simulink model "sudoku_PP_CEX2"  (R2017b)
settings: Solver=FixedStepDiscrete  StartTime=0.0  StopTime=10.0  FixedStep=0.200000  RelTol=1e-3
model workspace (MAT data in the model file):
  ContractValidatorBlocksMap = containers.Map
  ContractValidatorBlocksMap.serialization.keys = {'sudoku/contract/validator'}
  ContractValidatorBlocksMap.serialization.values{1}.block = 'sudoku/contract/validator'
  ContractValidatorBlocksMap.serialization.values{1}.assumePorts = 1
  ContractValidatorBlocksMap.serialization.values{1}.guaranteePorts = 1
  ContractValidatorBlocksMap.serialization.values{1}.modeBlocksPorts = 0
  ContractValidatorBlocksMap.serialization.values{1}.portHandles.Inport = [423.005737305 424.004150391]
  ContractValidatorBlocksMap.serialization.values{1}.portHandles.Outport = 425.013793945
  ContractValidatorBlocksMap.serialization.values{1}.portHandles.Enable = []
  ContractValidatorBlocksMap.serialization.values{1}.portHandles.Trigger = []
  ContractValidatorBlocksMap.serialization.values{1}.portHandles.State = []
  ContractValidatorBlocksMap.serialization.values{1}.portHandles.LConn = []
  ContractValidatorBlocksMap.serialization.values{1}.portHandles.RConn = []
  ContractValidatorBlocksMap.serialization.values{1}.portHandles.Ifaction = []
  ContractValidatorBlocksMap.serialization.values{1}.portHandles.Reset = []
  ContractValidatorBlocksMap.serialization.values{1}.portConnectivity(1).Type = '1'
  ContractValidatorBlocksMap.serialization.values{1}.portConnectivity(1).Position = [385 130]
  ContractValidatorBlocksMap.serialization.values{1}.portConnectivity(1).SrcBlock = 97.0111083984
  ContractValidatorBlocksMap.serialization.values{1}.portConnectivity(1).SrcPort = 0
  ContractValidatorBlocksMap.serialization.values{1}.portConnectivity(1).DstBlock = []
  ContractValidatorBlocksMap.serialization.values{1}.portConnectivity(1).DstPort = []
  ContractValidatorBlocksMap.serialization.values{1}.portConnectivity(2).Type = '2'
  ContractValidatorBlocksMap.serialization.values{1}.portConnectivity(2).Position = [385 270]
  ContractValidatorBlocksMap.serialization.values{1}.portConnectivity(2).SrcBlock = 134.024414062
  ContractValidatorBlocksMap.serialization.values{1}.portConnectivity(2).SrcPort = 0
  ContractValidatorBlocksMap.serialization.values{1}.portConnectivity(2).DstBlock = []
  ContractValidatorBlocksMap.serialization.values{1}.portConnectivity(2).DstPort = []
  ContractValidatorBlocksMap.serialization.values{1}.portConnectivity(3).Type = '1'
  ContractValidatorBlocksMap.serialization.values{1}.portConnectivity(3).Position = [500 200]
  ContractValidatorBlocksMap.serialization.values{1}.portConnectivity(3).SrcBlock = []
  ContractValidatorBlocksMap.serialization.values{1}.portConnectivity(3).SrcPort = []
  ContractValidatorBlocksMap.serialization.values{1}.portConnectivity(3).DstBlock = 409.010986328
  ContractValidatorBlocksMap.serialization.values{1}.portConnectivity(3).DstPort = 0
  ContractValidatorBlocksMap.serialization.uniformity = 0
  ContractValidatorBlocksMap.serialization.keyType = 'char'
  ContractValidatorBlocksMap.serialization.valueType = 'any'
  already_pp = 1
  compositionalMap.analysisNames = {'sudoku_PP/Sudoku'}
  compositionalMap.compositionalOptions = {{''}}
  compositionalMap.selectedOptions = 1
  maskControlsMap = containers.Map
  maskControlsMap.serialization.keys = {'sudoku_PP/contract/guarantee'}
  maskControlsMap.serialization.values = {{'Display_counter_example_as_signals', 'Display_counter_example_as_tables', 'Display_counter_example_as_HTML_tables', 'Generate_an_outer_model_for_the_counter_example', 'Generate_an_inner_model_for_the_counter_example'}}
  maskControlsMap.serialization.uniformity = 0
  maskControlsMap.serialization.keyType = 'char'
  maskControlsMap.serialization.valueType = 'any'
  nodeNameToBlockNameMap : containers.Map (value not decoded)
  verificationResults : struct (value not decoded)
undefined symbols (not defined in the file): contractAfterSimulation, ContractAssumeBlock, contractBeforeSimulation, ContractBlock, ContractGuaranteeBlock, ContractValidatorBlock, saveValidatorParameters
(part 1 of 17)
settings Model: Creator=hbourbou  LastModifiedBy=hbourbou
settings DebuggingCC: AlgebraicLoopMsg=error  ArtificialAlgebraicLoopMsg=error  SingleTaskRateTransMsg=error

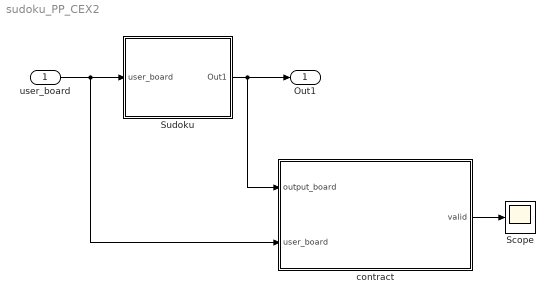
== system sudoku_PP_CEX2 ==
  user_board : Inport  OutDataTypeStr=uint8  PortDimensions=[9,9]
  Scope : Scope
  Sudoku : Subsystem  TreatAsAtomicUnit=on
  contract : Subsystem  TreatAsAtomicUnit=on  mask(ContractBlock){ContractBlockType=ContractBlock}
      mask init:
      | set_param(gcb, 'LinkStatus', 'none');
      settings: CopyFcn=set_param(gcb, 'LinkStatus', 'none');
      mask DialogControl DescTextVar Prompt: Contract block
      mask Display:
      | text(0.5, 0.5, '{\bf\fontsize{20}Contract}', 'hor', 'center', 'texmode','on');
      | blocks = find_system(gcb, 'LookUnderMasks','all', 'SearchDepth',1,'BlockType','Inport');
      | for i = 1 : length(blocks)
      |     blockName = get_param(blocks(i), 'Name');
      |     [path, blockName] = fileparts(char(blockName));
      |     port_label('input', i, blockName);
      | end
      | 
      | blocks = find_system(gcb, 'LookUnderMasks','all', 'SearchDepth',1,'BlockType','Outport');
      | for i = 1 : length(blocks)
      |     blockName = get_param(blocks(i), 'Name');
      |     [path, blockName] = fileparts(char(blockName));
      |     port_label('output', i, blockName);
      | end
  Out1 : Outport
  wires:
  Sudoku/1(Out1) -> contract/1(output_board), Out1/1
  user_board/1 -> contract/2(user_board), Sudoku/1(user_board)
  contract/1(valid) -> Scope/1

== system sudoku_PP_CEX2/Sudoku ==
  user_board : Inport
  Sum : Sum  Inputs=|++
  initial_board1 : Constant  Value=[0 0 0 0 0 0 0 0 0; 0 0 0 0 0 3 0 8 5; 0 0 1 0 2 0 0 0 0; 0 0 0 5 0 7 0 0 0; 0 0 4 0 0 0 1 0 0; 0 9 0 0 0 0 0 0 0; 5 0 0 0 0 0 0 7 3; 0 0 2 0 1 0 0 0 0; 0 0 0 0 4 0 0 0 9]  OutDataTypeStr=uint8
  Out1 : Outport
  wires:
  user_board/1 -> Sum/2
  initial_board1/1 -> Sum/1
  Sum/1 -> Out1/1

== system sudoku_PP_CEX2/contract ==
  output_board : Inport
  user_board : Inport  Port=2
  assume : Subsystem  TreatAsAtomicUnit=on  mask(ContractAssumeBlock){ContractBlockType=ContractAssumeBlock}
      mask init:
      | set_param(gcb, 'LinkStatus', 'none');
      mask DialogControl DescTextVar Prompt: Assume block
  guarantee : Subsystem  TreatAsAtomicUnit=on  mask(ContractGuaranteeBlock){ContractBlockType=ContractGuaranteeBlock}
      mask init:
      | set_param(gcb, 'LinkStatus', 'none');
      mask DialogControl DescTextVar Prompt: Guarantee block
      mask DialogControl Display_counter_example_as_signals Prompt: Display counter example as signals
      mask DialogControl Display_counter_example_as_signals Callback: displayCexSignals(1, 1);
      mask DialogControl Display_counter_example_as_tables Prompt: Display counter example as tables
      mask DialogControl Display_counter_example_as_tables Callback: displayCexTables(1, 1);
      mask DialogControl Display_counter_example_as_HTML_tables Prompt: Display counter example as HTML tables
      mask DialogControl Display_counter_example_as_HTML_tables Callback: displayCexHtmlTables(1, 1);
      mask DialogControl Generate_an_outer_model_for_the_counter_example Prompt: Generate an outer model for the counter example
      mask DialogControl Generate_an_outer_model_for_the_counter_example Callback: generateModelWithSignalBuilders(1, 1, 2);
      mask DialogControl Generate_an_inner_model_for_the_counter_example Prompt: Generate an inner model for the counter example
      mask DialogControl Generate_an_inner_model_for_the_counter_example Callback: generateModelWithSignalBuilders(1, 1, 1);
  validator : M-S-Function  LoadFcn=saveValidatorParameters(gcb);  InitFcn=contractBeforeSimulation();  StopFcn=contractAfterSimulation();  FunctionName=contract  mask(ContractValidatorBlock){assumePorts=1, guaranteePorts=1, modePorts=0, ContractBlockType=ContractValidatorBlock, createInportsCheckbox=off}
      mask prompts: assumePorts "Assume ports     :"; guaranteePorts "Guarantee ports :"; modePorts "Mode ports        :"; createInportsCheckbox "Create inports and connect them automatically"
      mask init:
      | set_param(gcb,'LinkStatus','none');
      | contract_callback('inputs_callback',gcb);
      mask DialogControl DescTextVar Prompt: The validator block implements the following logic: <br> <br> <b>Sofar</b>(assume<sub>1</sub> <b>&#8743;</b> assume<sub>2</sub> <b>&#8743;</b> ... assume<sub>k</sub>) <b>&rarr;</b> (guarantee<sub>1</sub> <b>&#8743;</b> guarantee<sub>2</sub> <b>&#8743;</b> ... guarantee<sub>m</sub> <b>&#8743;</b>  mode<sub>1</sub> <b>&#8743;</b> mode<sub>2</sub> <b>&#8743;</b> ... <b>&#8743;</b> mode<sub>n</sub> )<br> where mode<sub>i</sub> = require<sub>i</sub> <b>&rarr;</b> ensure<sub>i</sub>
      mask Display:
      | color('black');
      | port_label('input',1,'assume');
      | port_label('input',2,'guarantee');
      | port_label('output',1,'valid');
  valid : Outport
  wires:
  output_board/1 -> guarantee/1(Board)
  validator/1 -> valid/1
  guarantee/1(guarantee) -> validator/2
  assume/1(assume) -> validator/1
  user_board/1 -> assume/1(board)

== system sudoku_PP_CEX2/contract/assume ==
  board : Inport
  Element_minus_Wise_newline_Product : Product
  Logical_newline_Operator : Logic  Inputs=1  AllPortsSameDT=off  OutDataTypeStr=boolean
  Relational_newline_Operator : RelationalOperator  Operator===  OutDataTypeStr=boolean  RndMeth=Simplest
  Reshape : Reshape
  initial_board : Constant  Value=[0 0 0 0 0 0 0 0 0; 0 0 0 0 0 3 0 8 5; 0 0 1 0 2 0 0 0 0; 0 0 0 5 0 7 0 0 0; 0 0 4 0 0 0 1 0 0; 0 9 0 0 0 0 0 0 0; 5 0 0 0 0 0 0 7 3; 0 0 2 0 1 0 0 0 0; 0 0 0 0 4 0 0 0 9]  OutDataTypeStr=uint8
  zero : Constant  Value=zeros(9,9)  OutDataTypeStr=uint8
  assume : Outport  OutDataTypeStr=boolean
  wires:
  initial_board/1 -> Element_minus_Wise_newline_Product/1
  board/1 -> Element_minus_Wise_newline_Product/2
  Element_minus_Wise_newline_Product/1 -> Relational_newline_Operator/1
  zero/1 -> Relational_newline_Operator/2
  Relational_newline_Operator/1 -> Reshape/1
  Logical_newline_Operator/1 -> assume/1
  Reshape/1 -> Logical_newline_Operator/1

== system sudoku_PP_CEX2/contract/guarantee ==
  Board : Inport  PortDimensions=[9 9]
  BoxesValid : Subsystem  TreatAsAtomicUnit=on
  ColsValid : Subsystem  TreatAsAtomicUnit=on
  Logical_newline_Operator : Logic  Inputs=3  AllPortsSameDT=off  OutDataTypeStr=boolean
  Logical_newline_Operator1 : Logic  Operator=NOT  AllPortsSameDT=off  OutDataTypeStr=boolean
  RowsValid : Subsystem  TreatAsAtomicUnit=on
  guarantee : Outport  OutDataTypeStr=boolean
  wires:
  Board/1 -> BoxesValid/1(In1), RowsValid/1(In1), ColsValid/1(In1)
  RowsValid/1(Out1) -> Logical_newline_Operator/1
  ColsValid/1(Out1) -> Logical_newline_Operator/2
  BoxesValid/1(Out1) -> Logical_newline_Operator/3
  Logical_newline_Operator/1 -> Logical_newline_Operator1/1
  Logical_newline_Operator1/1 -> guarantee/1

== system sudoku_PP_CEX2/contract/guarantee/BoxesValid ==
  In1 : Inport
  ForEach_newline_Subsystem : Subsystem  TreatAsAtomicUnit=on
  Logical_newline_Operator : Logic  Inputs=1  AllPortsSameDT=off  OutDataTypeStr=boolean
  Out1 : Outport
  wires:
  In1/1 -> ForEach_newline_Subsystem/1(In1)
  ForEach_newline_Subsystem/1(Out1) -> Logical_newline_Operator/1
  Logical_newline_Operator/1 -> Out1/1

== system sudoku_PP_CEX2/contract/guarantee/ColsValid ==
  In1 : Inport
  ForEach_newline_Subsystem : Subsystem  TreatAsAtomicUnit=on
  Logical_newline_Operator : Logic  Inputs=1  AllPortsSameDT=off  OutDataTypeStr=boolean
  Out1 : Outport
  wires:
  In1/1 -> ForEach_newline_Subsystem/1(In1)
  ForEach_newline_Subsystem/1(Out1) -> Logical_newline_Operator/1
  Logical_newline_Operator/1 -> Out1/1

== system sudoku_PP_CEX2/contract/guarantee/RowsValid ==
  In1 : Inport
  ForEach_newline_Subsystem : Subsystem  TreatAsAtomicUnit=on
  Logical_newline_Operator : Logic  Inputs=1  AllPortsSameDT=off  OutDataTypeStr=boolean
  Out1 : Outport
  wires:
  In1/1 -> ForEach_newline_Subsystem/1(In1)
  ForEach_newline_Subsystem/1(Out1) -> Logical_newline_Operator/1
  Logical_newline_Operator/1 -> Out1/1

== system sudoku_PP_CEX2/contract/guarantee/BoxesValid/ForEach_newline_Subsystem ==
  In1 : Inport
  Concatenate_1 : Concatenate  NumInputs=3  Mode=Multidimensional array
  ForEach1 : Subsystem  TreatAsAtomicUnit=on
  ForEach2 : Subsystem  TreatAsAtomicUnit=on
  ForEach3 : Subsystem  TreatAsAtomicUnit=on
  Selector_1_In1 : Selector  NumberOfDimensions=2  IndexOptions=Index vector (dialog),Select all  Indices=[1 2 3],  OutputSizes=1
  Selector_2_In1 : Selector  NumberOfDimensions=2  IndexOptions=Index vector (dialog),Select all  Indices=[4 5 6],  OutputSizes=1
  Selector_3_In1 : Selector  NumberOfDimensions=2  IndexOptions=Index vector (dialog),Select all  Indices=[7 8 9],  OutputSizes=1
  Out1 : Outport
  wires:
  Concatenate_1/1 -> Out1/1
  Selector_3_In1/1 -> ForEach3/1(In1)
  Selector_2_In1/1 -> ForEach2/1(In1)
  Selector_1_In1/1 -> ForEach1/1(In1)
  ForEach3/1(Out1) -> Concatenate_1/3
  ForEach2/1(Out1) -> Concatenate_1/2
  ForEach1/1(Out1) -> Concatenate_1/1
  In1/1 -> Selector_3_In1/1, Selector_2_In1/1, Selector_1_In1/1

== system sudoku_PP_CEX2/contract/guarantee/ColsValid/ForEach_newline_Subsystem ==
  In1 : Inport
  Concatenate_1 : Concatenate  NumInputs=9  Mode=Multidimensional array
  ForEach1 : Subsystem  TreatAsAtomicUnit=on
  ForEach2 : Subsystem  TreatAsAtomicUnit=on
  ForEach3 : Subsystem  TreatAsAtomicUnit=on
  ForEach4 : Subsystem  TreatAsAtomicUnit=on
  ForEach5 : Subsystem  TreatAsAtomicUnit=on
  ForEach6 : Subsystem  TreatAsAtomicUnit=on
  ForEach7 : Subsystem  TreatAsAtomicUnit=on
  ForEach8 : Subsystem  TreatAsAtomicUnit=on
  ForEach9 : Subsystem  TreatAsAtomicUnit=on
  Selector_1_In1 : Selector  NumberOfDimensions=2  IndexOptions=Select all,Index vector (dialog)  Indices=,1  OutputSizes=1
  Selector_2_In1 : Selector  NumberOfDimensions=2  IndexOptions=Select all,Index vector (dialog)  Indices=,2  OutputSizes=1
  Selector_3_In1 : Selector  NumberOfDimensions=2  IndexOptions=Select all,Index vector (dialog)  Indices=,3  OutputSizes=1
  Selector_4_In1 : Selector  NumberOfDimensions=2  IndexOptions=Select all,Index vector (dialog)  Indices=,4  OutputSizes=1
  Selector_5_In1 : Selector  NumberOfDimensions=2  IndexOptions=Select all,Index vector (dialog)  Indices=,5  OutputSizes=1
  Selector_6_In1 : Selector  NumberOfDimensions=2  IndexOptions=Select all,Index vector (dialog)  Indices=,6  OutputSizes=1
  Selector_7_In1 : Selector  NumberOfDimensions=2  IndexOptions=Select all,Index vector (dialog)  Indices=,7  OutputSizes=1
  Selector_8_In1 : Selector  NumberOfDimensions=2  IndexOptions=Select all,Index vector (dialog)  Indices=,8  OutputSizes=1
  Selector_9_In1 : Selector  NumberOfDimensions=2  IndexOptions=Select all,Index vector (dialog)  Indices=,9  OutputSizes=1
  Out1 : Outport
  wires:
  Concatenate_1/1 -> Out1/1
  Selector_9_In1/1 -> ForEach9/1(In1)
  Selector_8_In1/1 -> ForEach8/1(In1)
  Selector_7_In1/1 -> ForEach7/1(In1)
  Selector_6_In1/1 -> ForEach6/1(In1)
  Selector_5_In1/1 -> ForEach5/1(In1)
  Selector_4_In1/1 -> ForEach4/1(In1)
  Selector_3_In1/1 -> ForEach3/1(In1)
  Selector_2_In1/1 -> ForEach2/1(In1)
  Selector_1_In1/1 -> ForEach1/1(In1)
  ForEach9/1(Out1) -> Concatenate_1/9
  ForEach8/1(Out1) -> Concatenate_1/8
  ForEach7/1(Out1) -> Concatenate_1/7
  ForEach6/1(Out1) -> Concatenate_1/6
  ForEach5/1(Out1) -> Concatenate_1/5
  ForEach4/1(Out1) -> Concatenate_1/4
  ForEach3/1(Out1) -> Concatenate_1/3
  ForEach2/1(Out1) -> Concatenate_1/2
  ForEach1/1(Out1) -> Concatenate_1/1
  In1/1 -> Selector_9_In1/1, Selector_8_In1/1, Selector_7_In1/1, Selector_6_In1/1, Selector_5_In1/1, Selector_4_In1/1, Selector_3_In1/1, Selector_2_In1/1, Selector_1_In1/1

== system sudoku_PP_CEX2/contract/guarantee/RowsValid/ForEach_newline_Subsystem ==
  In1 : Inport
  Concatenate_1 : Concatenate  NumInputs=9  Mode=Multidimensional array
  ForEach1 : Subsystem  TreatAsAtomicUnit=on
  ForEach2 : Subsystem  TreatAsAtomicUnit=on
  ForEach3 : Subsystem  TreatAsAtomicUnit=on
  ForEach4 : Subsystem  TreatAsAtomicUnit=on
  ForEach5 : Subsystem  TreatAsAtomicUnit=on
  ForEach6 : Subsystem  TreatAsAtomicUnit=on
  ForEach7 : Subsystem  TreatAsAtomicUnit=on
  ForEach8 : Subsystem  TreatAsAtomicUnit=on
  ForEach9 : Subsystem  TreatAsAtomicUnit=on
  Selector_1_In1 : Selector  NumberOfDimensions=2  IndexOptions=Index vector (dialog),Select all  Indices=1,  OutputSizes=1
  Selector_2_In1 : Selector  NumberOfDimensions=2  IndexOptions=Index vector (dialog),Select all  Indices=2,  OutputSizes=1
  Selector_3_In1 : Selector  NumberOfDimensions=2  IndexOptions=Index vector (dialog),Select all  Indices=3,  OutputSizes=1
  Selector_4_In1 : Selector  NumberOfDimensions=2  IndexOptions=Index vector (dialog),Select all  Indices=4,  OutputSizes=1
  Selector_5_In1 : Selector  NumberOfDimensions=2  IndexOptions=Index vector (dialog),Select all  Indices=5,  OutputSizes=1
  Selector_6_In1 : Selector  NumberOfDimensions=2  IndexOptions=Index vector (dialog),Select all  Indices=6,  OutputSizes=1
  Selector_7_In1 : Selector  NumberOfDimensions=2  IndexOptions=Index vector (dialog),Select all  Indices=7,  OutputSizes=1
  Selector_8_In1 : Selector  NumberOfDimensions=2  IndexOptions=Index vector (dialog),Select all  Indices=8,  OutputSizes=1
  Selector_9_In1 : Selector  NumberOfDimensions=2  IndexOptions=Index vector (dialog),Select all  Indices=9,  OutputSizes=1
  Out1 : Outport
  wires:
  Concatenate_1/1 -> Out1/1
  Selector_9_In1/1 -> ForEach9/1(In1)
  Selector_8_In1/1 -> ForEach8/1(In1)
  Selector_7_In1/1 -> ForEach7/1(In1)
  Selector_6_In1/1 -> ForEach6/1(In1)
  Selector_5_In1/1 -> ForEach5/1(In1)
  Selector_4_In1/1 -> ForEach4/1(In1)
  Selector_3_In1/1 -> ForEach3/1(In1)
  Selector_2_In1/1 -> ForEach2/1(In1)
  Selector_1_In1/1 -> ForEach1/1(In1)
  ForEach9/1(Out1) -> Concatenate_1/9
  ForEach8/1(Out1) -> Concatenate_1/8
  ForEach7/1(Out1) -> Concatenate_1/7
  ForEach6/1(Out1) -> Concatenate_1/6
  ForEach5/1(Out1) -> Concatenate_1/5
  ForEach4/1(Out1) -> Concatenate_1/4
  ForEach3/1(Out1) -> Concatenate_1/3
  ForEach2/1(Out1) -> Concatenate_1/2
  ForEach1/1(Out1) -> Concatenate_1/1
  In1/1 -> Selector_9_In1/1, Selector_8_In1/1, Selector_7_In1/1, Selector_6_In1/1, Selector_5_In1/1, Selector_4_In1/1, Selector_3_In1/1, Selector_2_In1/1, Selector_1_In1/1

== system sudoku_PP_CEX2/contract/guarantee/BoxesValid/ForEach_newline_Subsystem/ForEach1 ==
  In1 : Inport
  ForEach_newline_Subsystem : Subsystem  TreatAsAtomicUnit=on
  Logical_newline_Operator : Logic  Inputs=1  AllPortsSameDT=off  OutDataTypeStr=boolean
  Out1 : Outport
  wires:
  Logical_newline_Operator/1 -> Out1/1
  ForEach_newline_Subsystem/1(Out1) -> Logical_newline_Operator/1
  In1/1 -> ForEach_newline_Subsystem/1(In1)

== system sudoku_PP_CEX2/contract/guarantee/BoxesValid/ForEach_newline_Subsystem/ForEach2 ==
  In1 : Inport
  ForEach_newline_Subsystem : Subsystem  TreatAsAtomicUnit=on
  Logical_newline_Operator : Logic  Inputs=1  AllPortsSameDT=off  OutDataTypeStr=boolean
  Out1 : Outport
  wires:
  Logical_newline_Operator/1 -> Out1/1
  ForEach_newline_Subsystem/1(Out1) -> Logical_newline_Operator/1
  In1/1 -> ForEach_newline_Subsystem/1(In1)

== system sudoku_PP_CEX2/contract/guarantee/BoxesValid/ForEach_newline_Subsystem/ForEach3 ==
  In1 : Inport
  ForEach_newline_Subsystem : Subsystem  TreatAsAtomicUnit=on
  Logical_newline_Operator : Logic  Inputs=1  AllPortsSameDT=off  OutDataTypeStr=boolean
  Out1 : Outport
  wires:
  Logical_newline_Operator/1 -> Out1/1
  ForEach_newline_Subsystem/1(Out1) -> Logical_newline_Operator/1
  In1/1 -> ForEach_newline_Subsystem/1(In1)

== system sudoku_PP_CEX2/contract/guarantee/ColsValid/ForEach_newline_Subsystem/ForEach1 ==
  In1 : Inport
  Vectorisvalid : Subsystem  TreatAsAtomicUnit=on
  Out1 : Outport
  wires:
  Vectorisvalid/1(Out1) -> Out1/1
  In1/1 -> Vectorisvalid/1(In1)

== system sudoku_PP_CEX2/contract/guarantee/ColsValid/ForEach_newline_Subsystem/ForEach2 ==
  In1 : Inport
  Vectorisvalid : Subsystem  TreatAsAtomicUnit=on
  Out1 : Outport
  wires:
  Vectorisvalid/1(Out1) -> Out1/1
  In1/1 -> Vectorisvalid/1(In1)

== system sudoku_PP_CEX2/contract/guarantee/ColsValid/ForEach_newline_Subsystem/ForEach3 ==
  In1 : Inport
  Vectorisvalid : Subsystem  TreatAsAtomicUnit=on
  Out1 : Outport
  wires:
  Vectorisvalid/1(Out1) -> Out1/1
  In1/1 -> Vectorisvalid/1(In1)

== system sudoku_PP_CEX2/contract/guarantee/ColsValid/ForEach_newline_Subsystem/ForEach4 ==
  In1 : Inport
  Vectorisvalid : Subsystem  TreatAsAtomicUnit=on
  Out1 : Outport
  wires:
  Vectorisvalid/1(Out1) -> Out1/1
  In1/1 -> Vectorisvalid/1(In1)

== system sudoku_PP_CEX2/contract/guarantee/ColsValid/ForEach_newline_Subsystem/ForEach5 ==
  In1 : Inport
  Vectorisvalid : Subsystem  TreatAsAtomicUnit=on
  Out1 : Outport
  wires:
  Vectorisvalid/1(Out1) -> Out1/1
  In1/1 -> Vectorisvalid/1(In1)

== system sudoku_PP_CEX2/contract/guarantee/ColsValid/ForEach_newline_Subsystem/ForEach6 ==
  In1 : Inport
  Vectorisvalid : Subsystem  TreatAsAtomicUnit=on
  Out1 : Outport
  wires:
  Vectorisvalid/1(Out1) -> Out1/1
  In1/1 -> Vectorisvalid/1(In1)

== system sudoku_PP_CEX2/contract/guarantee/ColsValid/ForEach_newline_Subsystem/ForEach7 ==
  In1 : Inport
  Vectorisvalid : Subsystem  TreatAsAtomicUnit=on
  Out1 : Outport
  wires:
  Vectorisvalid/1(Out1) -> Out1/1
  In1/1 -> Vectorisvalid/1(In1)

== system sudoku_PP_CEX2/contract/guarantee/ColsValid/ForEach_newline_Subsystem/ForEach8 ==
  In1 : Inport
  Vectorisvalid : Subsystem  TreatAsAtomicUnit=on
  Out1 : Outport
  wires:
  Vectorisvalid/1(Out1) -> Out1/1
  In1/1 -> Vectorisvalid/1(In1)

== system sudoku_PP_CEX2/contract/guarantee/ColsValid/ForEach_newline_Subsystem/ForEach9 ==
  In1 : Inport
  Vectorisvalid : Subsystem  TreatAsAtomicUnit=on
  Out1 : Outport
  wires:
  Vectorisvalid/1(Out1) -> Out1/1
  In1/1 -> Vectorisvalid/1(In1)

== system sudoku_PP_CEX2/contract/guarantee/RowsValid/ForEach_newline_Subsystem/ForEach1 ==
  In1 : Inport
  Vectorisvalid : Subsystem  TreatAsAtomicUnit=on
  Out1 : Outport
  wires:
  Vectorisvalid/1(Out1) -> Out1/1
  In1/1 -> Vectorisvalid/1(In1)

== system sudoku_PP_CEX2/contract/guarantee/RowsValid/ForEach_newline_Subsystem/ForEach2 ==
  In1 : Inport
  Vectorisvalid : Subsystem  TreatAsAtomicUnit=on
  Out1 : Outport
  wires:
  Vectorisvalid/1(Out1) -> Out1/1
  In1/1 -> Vectorisvalid/1(In1)

== system sudoku_PP_CEX2/contract/guarantee/RowsValid/ForEach_newline_Subsystem/ForEach3 ==
  In1 : Inport
  Vectorisvalid : Subsystem  TreatAsAtomicUnit=on
  Out1 : Outport
  wires:
  Vectorisvalid/1(Out1) -> Out1/1
  In1/1 -> Vectorisvalid/1(In1)

== system sudoku_PP_CEX2/contract/guarantee/RowsValid/ForEach_newline_Subsystem/ForEach4 ==
  In1 : Inport
  Vectorisvalid : Subsystem  TreatAsAtomicUnit=on
  Out1 : Outport
  wires:
  Vectorisvalid/1(Out1) -> Out1/1
  In1/1 -> Vectorisvalid/1(In1)

== system sudoku_PP_CEX2/contract/guarantee/RowsValid/ForEach_newline_Subsystem/ForEach5 ==
  In1 : Inport
  Vectorisvalid : Subsystem  TreatAsAtomicUnit=on
  Out1 : Outport
  wires:
  Vectorisvalid/1(Out1) -> Out1/1
  In1/1 -> Vectorisvalid/1(In1)

== system sudoku_PP_CEX2/contract/guarantee/RowsValid/ForEach_newline_Subsystem/ForEach6 ==
  In1 : Inport
  Vectorisvalid : Subsystem  TreatAsAtomicUnit=on
  Out1 : Outport
  wires:
  Vectorisvalid/1(Out1) -> Out1/1
  In1/1 -> Vectorisvalid/1(In1)

== system sudoku_PP_CEX2/contract/guarantee/RowsValid/ForEach_newline_Subsystem/ForEach7 ==
  In1 : Inport
  Vectorisvalid : Subsystem  TreatAsAtomicUnit=on
  Out1 : Outport
  wires:
  Vectorisvalid/1(Out1) -> Out1/1
  In1/1 -> Vectorisvalid/1(In1)

== system sudoku_PP_CEX2/contract/guarantee/RowsValid/ForEach_newline_Subsystem/ForEach8 ==
  In1 : Inport
  Vectorisvalid : Subsystem  TreatAsAtomicUnit=on
  Out1 : Outport
  wires:
  Vectorisvalid/1(Out1) -> Out1/1
  In1/1 -> Vectorisvalid/1(In1)

== system sudoku_PP_CEX2/contract/guarantee/RowsValid/ForEach_newline_Subsystem/ForEach9 ==
  In1 : Inport
  Vectorisvalid : Subsystem  TreatAsAtomicUnit=on
  Out1 : Outport
  wires:
  Vectorisvalid/1(Out1) -> Out1/1
  In1/1 -> Vectorisvalid/1(In1)

== system sudoku_PP_CEX2/contract/guarantee/BoxesValid/ForEach_newline_Subsystem/ForEach1/ForEach_newline_Subsystem ==
  In1 : Inport
  Concatenate_1 : Concatenate  NumInputs=3  Mode=Multidimensional array
  ForEach1 : Subsystem  TreatAsAtomicUnit=on
  ForEach2 : Subsystem  TreatAsAtomicUnit=on
  ForEach3 : Subsystem  TreatAsAtomicUnit=on
  Selector_1_In1 : Selector  NumberOfDimensions=2  IndexOptions=Select all,Index vector (dialog)  Indices=,[1 2 3]  OutputSizes=1
  Selector_2_In1 : Selector  NumberOfDimensions=2  IndexOptions=Select all,Index vector (dialog)  Indices=,[4 5 6]  OutputSizes=1
  Selector_3_In1 : Selector  NumberOfDimensions=2  IndexOptions=Select all,Index vector (dialog)  Indices=,[7 8 9]  OutputSizes=1
  Out1 : Outport
  wires:
  Concatenate_1/1 -> Out1/1
  Selector_3_In1/1 -> ForEach3/1(In1)
  Selector_2_In1/1 -> ForEach2/1(In1)
  Selector_1_In1/1 -> ForEach1/1(In1)
  ForEach3/1(Out1) -> Concatenate_1/3
  ForEach2/1(Out1) -> Concatenate_1/2
  ForEach1/1(Out1) -> Concatenate_1/1
  In1/1 -> Selector_3_In1/1, Selector_2_In1/1, Selector_1_In1/1

== system sudoku_PP_CEX2/contract/guarantee/BoxesValid/ForEach_newline_Subsystem/ForEach2/ForEach_newline_Subsystem ==
  In1 : Inport
  Concatenate_1 : Concatenate  NumInputs=3  Mode=Multidimensional array
  ForEach1 : Subsystem  TreatAsAtomicUnit=on
  ForEach2 : Subsystem  TreatAsAtomicUnit=on
  ForEach3 : Subsystem  TreatAsAtomicUnit=on
  Selector_1_In1 : Selector  NumberOfDimensions=2  IndexOptions=Select all,Index vector (dialog)  Indices=,[1 2 3]  OutputSizes=1
  Selector_2_In1 : Selector  NumberOfDimensions=2  IndexOptions=Select all,Index vector (dialog)  Indices=,[4 5 6]  OutputSizes=1
  Selector_3_In1 : Selector  NumberOfDimensions=2  IndexOptions=Select all,Index vector (dialog)  Indices=,[7 8 9]  OutputSizes=1
  Out1 : Outport
  wires:
  Concatenate_1/1 -> Out1/1
  Selector_3_In1/1 -> ForEach3/1(In1)
  Selector_2_In1/1 -> ForEach2/1(In1)
  Selector_1_In1/1 -> ForEach1/1(In1)
  ForEach3/1(Out1) -> Concatenate_1/3
  ForEach2/1(Out1) -> Concatenate_1/2
  ForEach1/1(Out1) -> Concatenate_1/1
  In1/1 -> Selector_3_In1/1, Selector_2_In1/1, Selector_1_In1/1

== system sudoku_PP_CEX2/contract/guarantee/BoxesValid/ForEach_newline_Subsystem/ForEach3/ForEach_newline_Subsystem ==
  In1 : Inport
  Concatenate_1 : Concatenate  NumInputs=3  Mode=Multidimensional array
  ForEach1 : Subsystem  TreatAsAtomicUnit=on
  ForEach2 : Subsystem  TreatAsAtomicUnit=on
  ForEach3 : Subsystem  TreatAsAtomicUnit=on
  Selector_1_In1 : Selector  NumberOfDimensions=2  IndexOptions=Select all,Index vector (dialog)  Indices=,[1 2 3]  OutputSizes=1
  Selector_2_In1 : Selector  NumberOfDimensions=2  IndexOptions=Select all,Index vector (dialog)  Indices=,[4 5 6]  OutputSizes=1
  Selector_3_In1 : Selector  NumberOfDimensions=2  IndexOptions=Select all,Index vector (dialog)  Indices=,[7 8 9]  OutputSizes=1
  Out1 : Outport
  wires:
  Concatenate_1/1 -> Out1/1
  Selector_3_In1/1 -> ForEach3/1(In1)
  Selector_2_In1/1 -> ForEach2/1(In1)
  Selector_1_In1/1 -> ForEach1/1(In1)
  ForEach3/1(Out1) -> Concatenate_1/3
  ForEach2/1(Out1) -> Concatenate_1/2
  ForEach1/1(Out1) -> Concatenate_1/1
  In1/1 -> Selector_3_In1/1, Selector_2_In1/1, Selector_1_In1/1

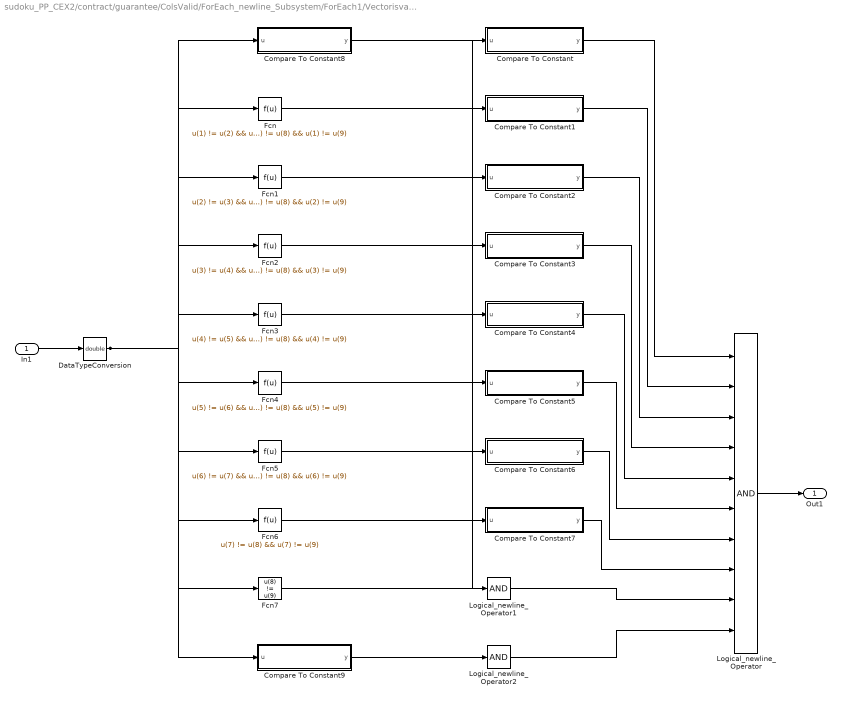
== system sudoku_PP_CEX2/contract/guarantee/ColsValid/ForEach_newline_Subsystem/ForEach1/Vectorisvalid ==
  In1 : Inport
  Compare To Constant : Subsystem  AncestorBlock=|  TreatAsAtomicUnit=on  mask(Compare To Constant){relop===, const=1, OutDataTypeStr=boolean, ZeroCross=on}
      | simulink/Logic and Bit
      | Operations/Compare
      | To Constant
      mask prompts: relop "Simulink:masks:Operator_MP"; const "Simulink:masks:ConstantValue_MP"; OutDataTypeStr "Simulink:masks:OutputDataType_MP"; ZeroCross "Simulink:masks:EnableZerocrossingDetection_MP"
      mask help: Simulink:masks:CompareToConstant_MD
      mask init:
      | blkName = gcb;
      | 
      | if strcmp(get_param(gcbh,'OutDataTypeStr'),'boolean')
      | 	setValue = 'boolean';
      | else
      | 	setValue = 'fixdt(0, 8)';
      | end
      | 
      | set_param([blkName,'/Compare'],'relop',relop, ...
      | 	'OutDataTypeStr', setValue, 'ZeroCross', ZeroCross);
      | 
      | str = [relop,' C']; %default
      | 
      | const_str = get_param(blkName, 'const');
      | const_val = str2num(const_str);
      | 
      | if isempty(const_val) %#ok<ST2NM>
      |     %Expression/Variable
      |     str = [relop, ' ', strtrim(const_str)];
      | else
      |     if length(const_val) == 1 
      |         if Simulink.data.isSupportedEnumClass(class(const_val))
      |             % Special Handling for Enumerations
      |             if Simulink.data.getEnumTypeInfo(class(const_val), 'AddClassNameToEnumNames')
      |                 str = [relop, ' ', strtrim(const_str)];
      |             else
      |                 str = [relop, ' ', char(const_val)];
      |             end
      |         elseif(isfloat(const_val) || isinteger(const_val) || islogical(const_val)) 
      |                 str = [relop, ' ', num2str(const_val)];
      |         end
      |     end
      | end
      mask TypeOptions relop: == | ~= | < | <= | >= | >
      mask TypeOptions OutDataTypeStr: Simulink:masks:uint8 | Simulink:masks:boolean
      mask Callback ZeroCross: sl('zeroCrossEnable', gcbh);
      mask Display: disp(str)
  Compare To Constant1 : Subsystem  AncestorBlock=|  TreatAsAtomicUnit=on  mask(Compare To Constant){relop===, const=1, OutDataTypeStr=boolean, ZeroCross=on}
      | simulink/Logic and Bit
      | Operations/Compare
      | To Constant
      mask prompts: relop "Simulink:masks:Operator_MP"; const "Simulink:masks:ConstantValue_MP"; OutDataTypeStr "Simulink:masks:OutputDataType_MP"; ZeroCross "Simulink:masks:EnableZerocrossingDetection_MP"
      mask help: Simulink:masks:CompareToConstant_MD
      mask init: same as sudoku_PP_CEX2/contract/guarantee/ColsValid/ForEach_newline_Subsystem/ForEach1/Vectorisvalid/Compare To Constant
      mask TypeOptions relop: == | ~= | < | <= | >= | >
      mask TypeOptions OutDataTypeStr: Simulink:masks:uint8 | Simulink:masks:boolean
      mask Callback ZeroCross: sl('zeroCrossEnable', gcbh);
      mask Display: disp(str)
  Compare To Constant2 : Subsystem  AncestorBlock=|  TreatAsAtomicUnit=on  mask(Compare To Constant){relop===, const=1, OutDataTypeStr=boolean, ZeroCross=on}
      | simulink/Logic and Bit
      | Operations/Compare
      | To Constant
      mask prompts: relop "Simulink:masks:Operator_MP"; const "Simulink:masks:ConstantValue_MP"; OutDataTypeStr "Simulink:masks:OutputDataType_MP"; ZeroCross "Simulink:masks:EnableZerocrossingDetection_MP"
      mask help: Simulink:masks:CompareToConstant_MD
      mask init: same as sudoku_PP_CEX2/contract/guarantee/ColsValid/ForEach_newline_Subsystem/ForEach1/Vectorisvalid/Compare To Constant
      mask TypeOptions relop: == | ~= | < | <= | >= | >
      mask TypeOptions OutDataTypeStr: Simulink:masks:uint8 | Simulink:masks:boolean
      mask Callback ZeroCross: sl('zeroCrossEnable', gcbh);
      mask Display: disp(str)
  Compare To Constant3 : Subsystem  AncestorBlock=|  TreatAsAtomicUnit=on  mask(Compare To Constant){relop===, const=1, OutDataTypeStr=boolean, ZeroCross=on}
      | simulink/Logic and Bit
      | Operations/Compare
      | To Constant
      mask prompts: relop "Simulink:masks:Operator_MP"; const "Simulink:masks:ConstantValue_MP"; OutDataTypeStr "Simulink:masks:OutputDataType_MP"; ZeroCross "Simulink:masks:EnableZerocrossingDetection_MP"
      mask help: Simulink:masks:CompareToConstant_MD
      mask init: same as sudoku_PP_CEX2/contract/guarantee/ColsValid/ForEach_newline_Subsystem/ForEach1/Vectorisvalid/Compare To Constant
      mask TypeOptions relop: == | ~= | < | <= | >= | >
      mask TypeOptions OutDataTypeStr: Simulink:masks:uint8 | Simulink:masks:boolean
      mask Callback ZeroCross: sl('zeroCrossEnable', gcbh);
      mask Display: disp(str)
  Compare To Constant4 : Subsystem  AncestorBlock=|  TreatAsAtomicUnit=on  mask(Compare To Constant){relop===, const=1, OutDataTypeStr=boolean, ZeroCross=on}
      | simulink/Logic and Bit
      | Operations/Compare
      | To Constant
      mask prompts: relop "Simulink:masks:Operator_MP"; const "Simulink:masks:ConstantValue_MP"; OutDataTypeStr "Simulink:masks:OutputDataType_MP"; ZeroCross "Simulink:masks:EnableZerocrossingDetection_MP"
      mask help: Simulink:masks:CompareToConstant_MD
      mask init: same as sudoku_PP_CEX2/contract/guarantee/ColsValid/ForEach_newline_Subsystem/ForEach1/Vectorisvalid/Compare To Constant
      mask TypeOptions relop: == | ~= | < | <= | >= | >
      mask TypeOptions OutDataTypeStr: Simulink:masks:uint8 | Simulink:masks:boolean
      mask Callback ZeroCross: sl('zeroCrossEnable', gcbh);
      mask Display: disp(str)
  Compare To Constant5 : Subsystem  AncestorBlock=|  TreatAsAtomicUnit=on  mask(Compare To Constant){relop===, const=1, OutDataTypeStr=boolean, ZeroCross=on}
      | simulink/Logic and Bit
      | Operations/Compare
      | To Constant
      mask prompts: relop "Simulink:masks:Operator_MP"; const "Simulink:masks:ConstantValue_MP"; OutDataTypeStr "Simulink:masks:OutputDataType_MP"; ZeroCross "Simulink:masks:EnableZerocrossingDetection_MP"
      mask help: Simulink:masks:CompareToConstant_MD
      mask init: same as sudoku_PP_CEX2/contract/guarantee/ColsValid/ForEach_newline_Subsystem/ForEach1/Vectorisvalid/Compare To Constant
      mask TypeOptions relop: == | ~= | < | <= | >= | >
      mask TypeOptions OutDataTypeStr: Simulink:masks:uint8 | Simulink:masks:boolean
      mask Callback ZeroCross: sl('zeroCrossEnable', gcbh);
      mask Display: disp(str)
  Compare To Constant6 : Subsystem  AncestorBlock=|  TreatAsAtomicUnit=on  mask(Compare To Constant){relop===, const=1, OutDataTypeStr=boolean, ZeroCross=on}
      | simulink/Logic and Bit
      | Operations/Compare
      | To Constant
      mask prompts: relop "Simulink:masks:Operator_MP"; const "Simulink:masks:ConstantValue_MP"; OutDataTypeStr "Simulink:masks:OutputDataType_MP"; ZeroCross "Simulink:masks:EnableZerocrossingDetection_MP"
      mask help: Simulink:masks:CompareToConstant_MD
      mask init: same as sudoku_PP_CEX2/contract/guarantee/ColsValid/ForEach_newline_Subsystem/ForEach1/Vectorisvalid/Compare To Constant
      mask TypeOptions relop: == | ~= | < | <= | >= | >
      mask TypeOptions OutDataTypeStr: Simulink:masks:uint8 | Simulink:masks:boolean
      mask Callback ZeroCross: sl('zeroCrossEnable', gcbh);
      mask Display: disp(str)
  Compare To Constant7 : Subsystem  AncestorBlock=|  TreatAsAtomicUnit=on  mask(Compare To Constant){relop===, const=1, OutDataTypeStr=boolean, ZeroCross=on}
      | simulink/Logic and Bit
      | Operations/Compare
      | To Constant
      mask prompts: relop "Simulink:masks:Operator_MP"; const "Simulink:masks:ConstantValue_MP"; OutDataTypeStr "Simulink:masks:OutputDataType_MP"; ZeroCross "Simulink:masks:EnableZerocrossingDetection_MP"
      mask help: Simulink:masks:CompareToConstant_MD
      mask init: same as sudoku_PP_CEX2/contract/guarantee/ColsValid/ForEach_newline_Subsystem/ForEach1/Vectorisvalid/Compare To Constant
      mask TypeOptions relop: == | ~= | < | <= | >= | >
      mask TypeOptions OutDataTypeStr: Simulink:masks:uint8 | Simulink:masks:boolean
      mask Callback ZeroCross: sl('zeroCrossEnable', gcbh);
      mask Display: disp(str)
  Compare To Constant8 : Subsystem  AncestorBlock=|  TreatAsAtomicUnit=on  mask(Compare To Constant){relop=>=, const=1, OutDataTypeStr=boolean, ZeroCross=on}
      | simulink/Logic and Bit
      | Operations/Compare
      | To Constant
      mask prompts: relop "Simulink:masks:Operator_MP"; const "Simulink:masks:ConstantValue_MP"; OutDataTypeStr "Simulink:masks:OutputDataType_MP"; ZeroCross "Simulink:masks:EnableZerocrossingDetection_MP"
      mask help: Simulink:masks:CompareToConstant_MD
      mask init: same as sudoku_PP_CEX2/contract/guarantee/ColsValid/ForEach_newline_Subsystem/ForEach1/Vectorisvalid/Compare To Constant
      mask TypeOptions relop: == | ~= | < | <= | >= | >
      mask TypeOptions OutDataTypeStr: Simulink:masks:uint8 | Simulink:masks:boolean
      mask Callback ZeroCross: sl('zeroCrossEnable', gcbh);
      mask Display: disp(str)
  Compare To Constant9 : Subsystem  AncestorBlock=|  TreatAsAtomicUnit=on  mask(Compare To Constant){relop=<=, const=9, OutDataTypeStr=boolean, ZeroCross=on}
      | simulink/Logic and Bit
      | Operations/Compare
      | To Constant
      mask prompts: relop "Simulink:masks:Operator_MP"; const "Simulink:masks:ConstantValue_MP"; OutDataTypeStr "Simulink:masks:OutputDataType_MP"; ZeroCross "Simulink:masks:EnableZerocrossingDetection_MP"
      mask help: Simulink:masks:CompareToConstant_MD
      mask init: same as sudoku_PP_CEX2/contract/guarantee/ColsValid/ForEach_newline_Subsystem/ForEach1/Vectorisvalid/Compare To Constant
      mask TypeOptions relop: == | ~= | < | <= | >= | >
      mask TypeOptions OutDataTypeStr: Simulink:masks:uint8 | Simulink:masks:boolean
      mask Callback ZeroCross: sl('zeroCrossEnable', gcbh);
      mask Display: disp(str)
  DataTypeConversion : DataTypeConversion  OutDataTypeStr=double
  Fcn : Fcn  Expr=u(1) != u(2) && u(1) != u(3) && u(1) != u(4) && u(1) != u(5) && u(1) != u(6) && u(1) != u(7) && u(1) != u(8) && u(1) != u(9)
  Fcn1 : Fcn  Expr=u(2) != u(3) && u(2) != u(4) && u(2) != u(5) && u(2) != u(6) && u(2) != u(7) && u(2) != u(8) && u(2) != u(9)
  Fcn2 : Fcn  Expr=u(3) != u(4) && u(3) != u(5) && u(3) != u(6) && u(3) != u(7) && u(3) != u(8) && u(3) != u(9)
  Fcn3 : Fcn  Expr=u(4) != u(5) && u(4) != u(6) && u(4) != u(7) && u(4) != u(8) && u(4) != u(9)
  Fcn4 : Fcn  Expr=u(5) != u(6) && u(5) != u(7) && u(5) != u(8) && u(5) != u(9)
  Fcn5 : Fcn  Expr=u(6) != u(7) && u(6) != u(8) && u(6) != u(9)
  Fcn6 : Fcn  Expr=u(7) != u(8) && u(7) != u(9)
  Fcn7 : Fcn  Expr=u(8) != u(9)
  Logical_newline_Operator : Logic  Inputs=10  AllPortsSameDT=off  OutDataTypeStr=boolean
  Logical_newline_Operator1 : Logic  Inputs=1  AllPortsSameDT=off  OutDataTypeStr=boolean
  Logical_newline_Operator2 : Logic  Inputs=1  AllPortsSameDT=off  OutDataTypeStr=boolean
  Out1 : Outport
  wires:
  Logical_newline_Operator/1 -> Out1/1
  Compare To Constant9/1(y) -> Logical_newline_Operator2/1
  Compare To Constant8/1(y) -> Logical_newline_Operator1/1
  Logical_newline_Operator2/1 -> Logical_newline_Operator/10
  Logical_newline_Operator1/1 -> Logical_newline_Operator/9
  Compare To Constant7/1(y) -> Logical_newline_Operator/8
  Compare To Constant6/1(y) -> Logical_newline_Operator/7
  Compare To Constant5/1(y) -> Logical_newline_Operator/6
  Compare To Constant4/1(y) -> Logical_newline_Operator/5
  Compare To Constant3/1(y) -> Logical_newline_Operator/4
  Compare To Constant2/1(y) -> Logical_newline_Operator/3
  Compare To Constant1/1(y) -> Logical_newline_Operator/2
  Compare To Constant/1(y) -> Logical_newline_Operator/1
  In1/1 -> DataTypeConversion/1
  Fcn7/1 -> Compare To Constant7/1(u)
  Fcn6/1 -> Compare To Constant6/1(u)
  Fcn5/1 -> Compare To Constant5/1(u)
  Fcn4/1 -> Compare To Constant4/1(u)
  Fcn3/1 -> Compare To Constant3/1(u)
  Fcn2/1 -> Compare To Constant2/1(u)
  Fcn1/1 -> Compare To Constant1/1(u)
  Fcn/1 -> Compare To Constant/1(u)
  DataTypeConversion/1 -> Fcn7/1, Fcn6/1, Fcn5/1, Fcn4/1, Fcn3/1, Fcn2/1, Fcn1/1, Fcn/1, Compare To Constant9/1(u), Compare To Constant8/1(u)
